simulink model "model_for_figure (EEE-13255's conflicted copy 2017-08-23)"  (R2016b)
settings: Solver=VariableStepAuto  StartTime=0.0  StopTime=5000  RelTol=1e-3
undefined symbols (not defined in the file or in its folder): sigbuilder_block
settings Model: Creator=utomo  LastModifiedBy=utomo

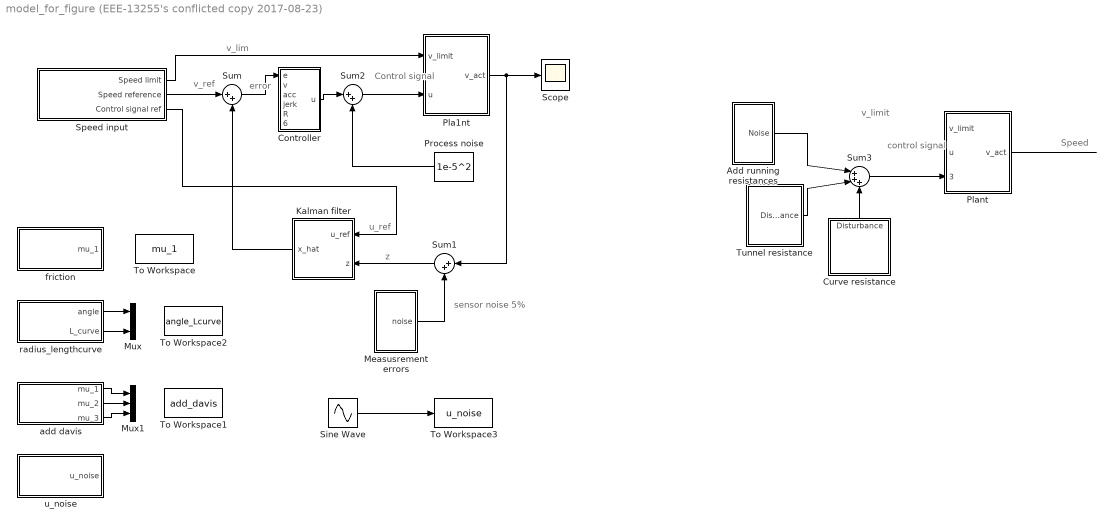
== system model_for_figure (EEE-13255's conflicted copy 2017-08-23) ==
  note: Speed
  note: control
      | signal
  note: v_limit
  note: sensor noise
      | 5%
  note: z
  note: error
  note: v_lim
  note: v_ref
  note: Control
      | signal
  note: u_ref
  Add running resistances : Subsystem
  Controller : Subsystem
  Curve resistance : Subsystem
  Kalman filter : Subsystem
  Measusrement errors : Subsystem
  Mux : Mux  Inputs=2
  Mux1 : Mux  Inputs=3
  Pla1nt : Subsystem
  Plant : Subsystem
  Process noise : Constant  Value=1e-5^2
  Scope : Scope
  Sine Wave : Sin  Amplitude=1e-5^2  Frequency=1/100  SampleTime=1
  Speed input : Subsystem  Tag=STV Subsys  LoadFcn=sigbuilder_block('load');  StartFcn=sigbuilder_block('start');  StopFcn=sigbuilder_block('stop');  ClipboardFcn=sigbuilder_block('clipboard');  mask(Sigbuilder block){tuvar=[0:10]}
      mask help: Simulink:masks:SigbuilderBlock_MD
      mask init:
      | if ~strcmp(get_param(bdroot(gcbh),'SimulationStatus'),'stopped') tuvar = sigbuilder_block('maskInit'); end
      settings: CopyFcn=sigbuilder_block('copy');  DeleteFcn=sigbuilder_block('delete');  ModelCloseFcn=sigbuilder_block('modelClose');  PreSaveFcn=sigbuilder_block('preSave');  PauseFcn=sigbuilder_block('pause');  ContinueFcn=sigbuilder_block('continue');  NameChangeFcn=sigbuilder_block('namechange');  OpenFcn=sigbuilder_block('open',[437.25 153 550.5 359.25 ]);  CloseFcn=sigbuilder_block('close');
      mask Display: plot(0, 0, 100, 100,[2, 2, 32, 32, 2], [68, 8, 8, 68, 68],[32, 2], [38, 38], [32, 19, 2],[53, 60, 44], [32, 17, 17, 2],[16, 16, 31, 31]);txt = getActiveGroup(gcbh);text(2, 100, txt,'verticalAlignment', 'top');
  Sum : Sum  Inputs=|++
  Sum1 : Sum  Inputs=|++
  Sum2 : Sum  Inputs=|++
  Sum3 : Sum  Inputs=|+++
  To Workspace : ToWorkspace  VariableName=mu_1  SampleTime=1
      settings: Save2DSignal=2-D array (concatenate along first dimension)
  To Workspace1 : ToWorkspace  VariableName=add_davis  SampleTime=1
      settings: Save2DSignal=2-D array (concatenate along first dimension)
  To Workspace2 : ToWorkspace  VariableName=angle_Lcurve  SampleTime=1
      settings: Save2DSignal=2-D array (concatenate along first dimension)
  To Workspace3 : ToWorkspace  VariableName=u_noise  SampleTime=1
      settings: Save2DSignal=2-D array (concatenate along first dimension)
  Tunnel resistance : Subsystem
  add davis : Subsystem  Tag=STV Subsys  LoadFcn=sigbuilder_block('load');  StartFcn=sigbuilder_block('start');  StopFcn=sigbuilder_block('stop');  ClipboardFcn=sigbuilder_block('clipboard');  mask(Sigbuilder block){tuvar=[0:10]}
      mask help: Simulink:masks:SigbuilderBlock_MD
      mask init:
      | if ~strcmp(get_param(bdroot(gcbh),'SimulationStatus'),'stopped') tuvar = sigbuilder_block('maskInit'); end
      settings: CopyFcn=sigbuilder_block('copy');  DeleteFcn=sigbuilder_block('delete');  ModelCloseFcn=sigbuilder_block('modelClose');  PreSaveFcn=sigbuilder_block('preSave');  PauseFcn=sigbuilder_block('pause');  ContinueFcn=sigbuilder_block('continue');  NameChangeFcn=sigbuilder_block('namechange');  OpenFcn=sigbuilder_block('open',[437.25 153 550.5 359.25 ]);  CloseFcn=sigbuilder_block('close');
      mask Display: plot(0, 0, 100, 100,[2, 2, 32, 32, 2], [68, 8, 8, 68, 68],[32, 2], [38, 38], [32, 19, 2],[53, 60, 44], [32, 17, 17, 2],[16, 16, 31, 31]);txt = getActiveGroup(gcbh);text(2, 100, txt,'verticalAlignment', 'top');
  "friction " : Subsystem  Tag=STV Subsys  LoadFcn=sigbuilder_block('load');  StartFcn=sigbuilder_block('start');  StopFcn=sigbuilder_block('stop');  ClipboardFcn=sigbuilder_block('clipboard');  mask(Sigbuilder block){tuvar=[0:10]}
      mask help: Simulink:masks:SigbuilderBlock_MD
      mask init:
      | if ~strcmp(get_param(bdroot(gcbh),'SimulationStatus'),'stopped') tuvar = sigbuilder_block('maskInit'); end
      settings: CopyFcn=sigbuilder_block('copy');  DeleteFcn=sigbuilder_block('delete');  ModelCloseFcn=sigbuilder_block('modelClose');  PreSaveFcn=sigbuilder_block('preSave');  PauseFcn=sigbuilder_block('pause');  ContinueFcn=sigbuilder_block('continue');  NameChangeFcn=sigbuilder_block('namechange');  OpenFcn=sigbuilder_block('open',[437.25 153 550.5 359.25 ]);  CloseFcn=sigbuilder_block('close');
      mask Display: plot(0, 0, 100, 100,[2, 2, 32, 32, 2], [68, 8, 8, 68, 68],[32, 2], [38, 38], [32, 19, 2],[53, 60, 44], [32, 17, 17, 2],[16, 16, 31, 31]);txt = getActiveGroup(gcbh);text(2, 100, txt,'verticalAlignment', 'top');
  radius_lengthcurve : Subsystem  Tag=STV Subsys  LoadFcn=sigbuilder_block('load');  StartFcn=sigbuilder_block('start');  StopFcn=sigbuilder_block('stop');  ClipboardFcn=sigbuilder_block('clipboard');  mask(Sigbuilder block){tuvar=[0:10]}
      mask help: Simulink:masks:SigbuilderBlock_MD
      mask init:
      | if ~strcmp(get_param(bdroot(gcbh),'SimulationStatus'),'stopped') tuvar = sigbuilder_block('maskInit'); end
      settings: CopyFcn=sigbuilder_block('copy');  DeleteFcn=sigbuilder_block('delete');  ModelCloseFcn=sigbuilder_block('modelClose');  PreSaveFcn=sigbuilder_block('preSave');  PauseFcn=sigbuilder_block('pause');  ContinueFcn=sigbuilder_block('continue');  NameChangeFcn=sigbuilder_block('namechange');  OpenFcn=sigbuilder_block('open',[416.25 111.75 550.5 359.25 ]);  CloseFcn=sigbuilder_block('close');
      mask Display: plot(0, 0, 100, 100,[2, 2, 32, 32, 2], [68, 8, 8, 68, 68],[32, 2], [38, 38], [32, 19, 2],[53, 60, 44], [32, 17, 17, 2],[16, 16, 31, 31]);txt = getActiveGroup(gcbh);text(2, 100, txt,'verticalAlignment', 'top');
  u_noise : Subsystem  Tag=STV Subsys  LoadFcn=sigbuilder_block('load');  StartFcn=sigbuilder_block('start');  StopFcn=sigbuilder_block('stop');  ClipboardFcn=sigbuilder_block('clipboard');  mask(Sigbuilder block){tuvar=[0:10]}
      mask help: Simulink:masks:SigbuilderBlock_MD
      mask init:
      | if ~strcmp(get_param(bdroot(gcbh),'SimulationStatus'),'stopped') tuvar = sigbuilder_block('maskInit'); end
      settings: CopyFcn=sigbuilder_block('copy');  DeleteFcn=sigbuilder_block('delete');  ModelCloseFcn=sigbuilder_block('modelClose');  PreSaveFcn=sigbuilder_block('preSave');  PauseFcn=sigbuilder_block('pause');  ContinueFcn=sigbuilder_block('continue');  NameChangeFcn=sigbuilder_block('namechange');  OpenFcn=sigbuilder_block('open',[437.25 153 550.5 359.25 ]);  CloseFcn=sigbuilder_block('close');
      mask Display: plot(0, 0, 100, 100,[2, 2, 32, 32, 2], [68, 8, 8, 68, 68],[32, 2], [38, 38], [32, 19, 2],[53, 60, 44], [32, 17, 17, 2],[16, 16, 31, 31]);txt = getActiveGroup(gcbh);text(2, 100, txt,'verticalAlignment', 'top');
  wires:
  Sum/1 -> Controller/1(e)
  Speed input/2(Speed reference) -> Sum/1
  Speed input/1(Speed limit) -> Pla1nt/1(v_limit)
  Pla1nt/1(v_act) -> Sum1/1, Scope/1
  Measusrement errors/1(noise) -> Sum1/2
  Sum1/1 -> Kalman filter/2(z)
  Kalman filter/1(x_hat) -> Sum/2
  Speed input/3(Control signal ref) -> Kalman filter/1(u_ref)
  Controller/1(u) -> Sum2/1
  Sum2/1 -> Pla1nt/2(u)
  Process noise/1 -> Sum2/2
  radius_lengthcurve/1(angle) -> Mux/1
  radius_lengthcurve/2(L_curve) -> Mux/2
  add davis/2(mu_2) -> Mux1/2
  add davis/3(mu_3) -> Mux1/3
  add davis/1(mu_1) -> Mux1/1
  Sine Wave/1 -> To Workspace3/1
  Sum3/1 -> Plant/3(disturbances)
  Add running resistances/1(Noise) -> Sum3/1
  Tunnel resistance/1(Disturbance) -> Sum3/2
  Curve resistance/1(Disturbance) -> Sum3/3
  ? -> Plant/1(v_limit)
  ? -> Plant/2(u)
  Plant/1(v_act) -> ?

== system model_for_figure (EEE-13255's conflicted copy 2017-08-23)/Add running resistances ==
  Gain : Gain
  Noise : Outport
  wires:
  ? -> Gain/1
  Gain/1 -> Noise/1

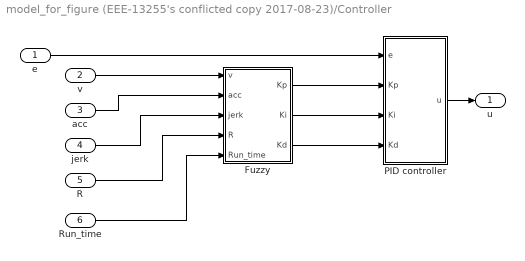
== system model_for_figure (EEE-13255's conflicted copy 2017-08-23)/Controller ==
  e : Inport
  v : Inport  Port=2
  acc : Inport  Port=3
  jerk : Inport  Port=4
  R : Inport  Port=5
  Run_time : Inport  Port=6
  Fuzzy : Subsystem
  PID controller : Subsystem
  u : Outport
  wires:
  e/1 -> PID controller/1(e)
  PID controller/1(u) -> u/1
  Fuzzy/1(Kp) -> PID controller/2(Kp)
  Fuzzy/2(Ki) -> PID controller/3(Ki)
  Fuzzy/3(Kd) -> PID controller/4(Kd)
  v/1 -> Fuzzy/1(v)
  acc/1 -> Fuzzy/2(acc)
  jerk/1 -> Fuzzy/3(jerk)
  R/1 -> Fuzzy/4(R)
  Run_time/1 -> Fuzzy/5(Run_time)

== system model_for_figure (EEE-13255's conflicted copy 2017-08-23)/Curve resistance ==
  Gain : Gain
  Disturbance : Outport
  wires:
  ? -> Gain/1
  Gain/1 -> Disturbance/1

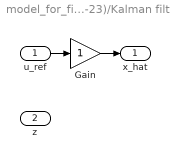
== system model_for_figure (EEE-13255's conflicted copy 2017-08-23)/Kalman filter ==
  u_ref : Inport
  z : Inport  Port=2
  Gain : Gain
  x_hat : Outport
  wires:
  u_ref/1 -> Gain/1
  Gain/1 -> x_hat/1

== system model_for_figure (EEE-13255's conflicted copy 2017-08-23)/Measusrement errors ==
  Gain : Gain
  noise : Outport
  wires:
  Gain/1 -> noise/1
  ? -> Gain/1

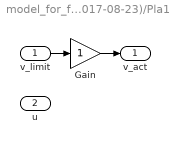
== system model_for_figure (EEE-13255's conflicted copy 2017-08-23)/Pla1nt ==
  v_limit : Inport
  u : Inport  Port=2
  Gain : Gain
  v_act : Outport
  wires:
  v_limit/1 -> Gain/1
  Gain/1 -> v_act/1

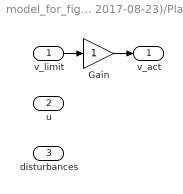
== system model_for_figure (EEE-13255's conflicted copy 2017-08-23)/Plant ==
  v_limit : Inport
  u : Inport  Port=2
  disturbances : Inport  Port=3
  Gain : Gain
  v_act : Outport
  wires:
  Gain/1 -> v_act/1
  v_limit/1 -> Gain/1

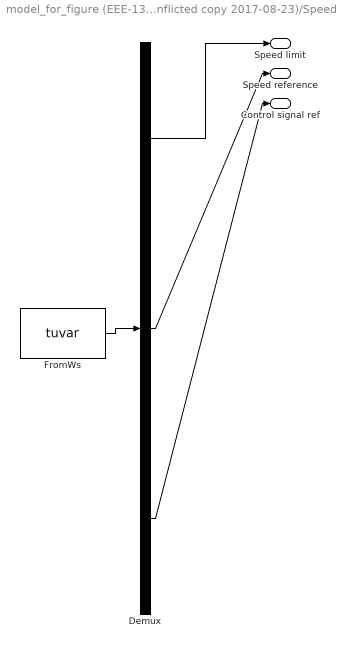
== system model_for_figure (EEE-13255's conflicted copy 2017-08-23)/Speed input ==
  Demux : Demux  Tag=STV Demux  Outputs=3
  FromWs : FromWorkspace  Tag=STV FromWs  VariableName=tuvar  SampleTime=0
      SigBuilderData=|
      | common.afterFinalStr = 'Extrapolate'
      | common.sampleTime = 0
      | dataSet.timeRange = [0 10]
      | dataSet.name = 'Group 1'
      | sbobj.Groups.Name = 'Group 1'
      | sbobj.Groups.Signals(1).Name = 'Speed limit'
      | sbobj.Groups.Signals(1).XData = [0 4 4 6 6 10]
      | sbobj.Groups.Signals(1).YData = [0 0 1 1 0 0]
      | sbobj.Groups.Signals(2).Name = 'Speed reference'
      | sbobj.Groups.Signals(2).XData = [0 10]
      | sbobj.Groups.Signals(2).YData = [0 0]
      | sbobj.Groups.Signals(3).Name = 'Control signal ref'
      | sbobj.Groups.Signals(3).XData = [0 10]
      | sbobj.Groups.Signals(3).YData = [0 0]
  Speed limit : Outport  Tag=STV Outport
  Speed reference : Outport  Tag=STV Outport  Port=2
  Control signal ref : Outport  Tag=STV Outport  Port=3
  wires:
  Demux/1 -> Speed limit/1
  FromWs/1 -> Demux/1
  Demux/2 -> Speed reference/1
  Demux/3 -> Control signal ref/1

== system model_for_figure (EEE-13255's conflicted copy 2017-08-23)/Tunnel resistance ==
  Gain : Gain
  Disturbance : Outport
  wires:
  Gain/1 -> Disturbance/1
  ? -> Gain/1

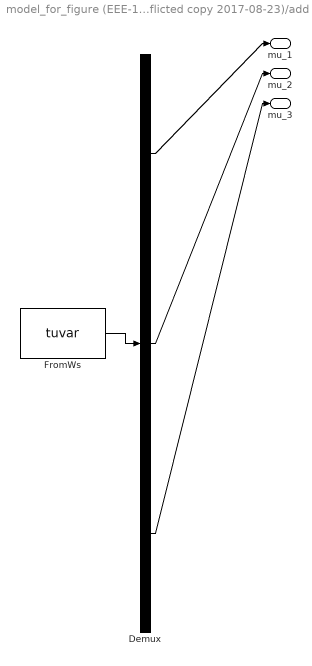
== system model_for_figure (EEE-13255's conflicted copy 2017-08-23)/add davis ==
  Demux : Demux  Tag=STV Demux  Outputs=3
  FromWs : FromWorkspace  Tag=STV FromWs  VariableName=tuvar
      SigBuilderData=|
      | common.afterFinalStr = 'Extrapolate'
      | common.sampleTime = '-1'
      | dataSet.timeRange = [0 5000]
      | dataSet.name = 'Group 1'
      | sbobj.Groups.Name = 'Group 1'
      | sbobj.Groups.Signals(1).Name = 'mu_1'
      | sbobj.Groups.Signals(1).XData = [0 500 500 1000 1500 2000 2000 2500 3000 3500 4000 4500 5000]
      | sbobj.Groups.Signals(1).YData = [1 0.7 0.9 1.1 1 1.2 0.8 0.9 0.9 1.1 1.05 0.9 1.1]
      | sbobj.Groups.Signals(2).Name = 'mu_2'
      | sbobj.Groups.Signals(2).XData = [0 500 500 1000 1500 2000 2000 2500 3000 3500 4000 4500 5000]
      | sbobj.Groups.Signals(2).YData = [0.9 1 0.9 1 0.8 1 1.1 0.7 1.2 0.9 1 1.1 0.9]
      | sbobj.Groups.Signals(3).Name = 'mu_3'
      | sbobj.Groups.Signals(3).XData = [0 500 500 1000 1500 2000 2000 2500 3000 3500 4000 4500 5000]
      | sbobj.Groups.Signals(3).YData = [0.7 0.8 1 0.8 1.1 0.8 1 1.05 1.1 1.2 0.8 0.9 0.99]
      | sbobj.Groups.TimeRange = [0 5000]
  mu_1 : Outport  Tag=STV Outport
  mu_2 : Outport  Tag=STV Outport  Port=2
  mu_3 : Outport  Tag=STV Outport  Port=3
  wires:
  Demux/1 -> mu_1/1
  FromWs/1 -> Demux/1
  Demux/2 -> mu_2/1
  Demux/3 -> mu_3/1

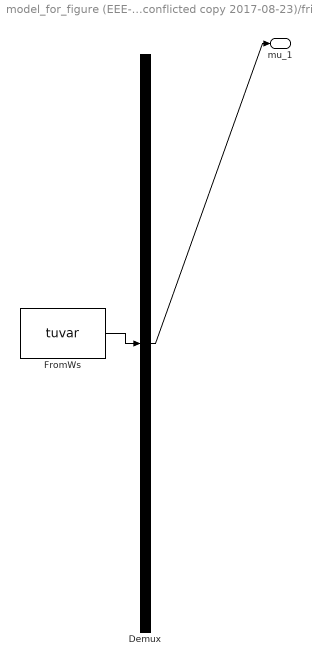
== system model_for_figure (EEE-13255's conflicted copy 2017-08-23)/friction  ==
  Demux : Demux  Tag=STV Demux  Outputs=1
  FromWs : FromWorkspace  Tag=STV FromWs  VariableName=tuvar
      SigBuilderData=|
      | common.afterFinalStr = 'Extrapolate'
      | common.sampleTime = '-1'
      | dataSet.timeRange = [0 5000]
      | dataSet.name = 'Group 1'
      | sbobj.Groups.Name = 'Group 1'
      | sbobj.Groups.Signals.Name = 'mu_1'
      | sbobj.Groups.Signals.XData = [0 3.24 500 1000 1500 2000 2000 2500 3000 3500 4000 4500 5000]
      | sbobj.Groups.Signals.YData = [0 0 0.1 0.385 0.6 0.25 0.05 0.305 0.9 0.8 0.7 0.2 0.499401197605]
      | sbobj.Groups.TimeRange = [0 5000]
  mu_1 : Outport  Tag=STV Outport
  wires:
  FromWs/1 -> Demux/1
  Demux/1 -> mu_1/1

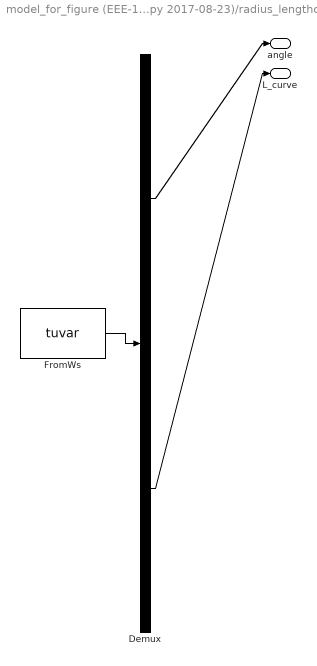
== system model_for_figure (EEE-13255's conflicted copy 2017-08-23)/radius_lengthcurve ==
  Demux : Demux  Tag=STV Demux  Outputs=2
  FromWs : FromWorkspace  Tag=STV FromWs  VariableName=tuvar
      SigBuilderData=|
      | common.afterFinalStr = 'Extrapolate'
      | common.sampleTime = '-1'
      | dataSet.timeRange = [0 5000]
      | dataSet.name = 'Group 1'
      | sbobj.Groups.Name = 'Group 1'
      | sbobj.Groups.Signals(1).Name = 'angle'
      | sbobj.Groups.Signals(1).XData = [0 3.24 101 101 300 300 3001 3001 4000 4000 4401 4401 4900 4900 5000]
      | sbobj.Groups.Signals(1).YData = [0 0 0 90 90 0 0 190 190 0 0 75 75 0 0]
      | sbobj.Groups.Signals(2).Name = 'L_curve'
      | sbobj.Groups.Signals(2).XData = [0 3.24 101 101 300 300 3001 3001 4000 4000 4401 4401 4900 4900 5000]
      | sbobj.Groups.Signals(2).YData = [0 0 0 200 200 0 0 1000 1000 0 0 500 500 0 0]
      | sbobj.Groups.TimeRange = [0 5000]
  angle : Outport  Tag=STV Outport
  L_curve : Outport  Tag=STV Outport  Port=2
  wires:
  Demux/1 -> angle/1
  FromWs/1 -> Demux/1
  Demux/2 -> L_curve/1

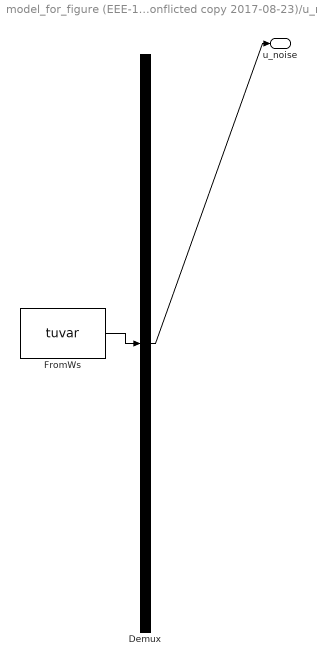
== system model_for_figure (EEE-13255's conflicted copy 2017-08-23)/u_noise ==
  Demux : Demux  Tag=STV Demux  Outputs=1
  FromWs : FromWorkspace  Tag=STV FromWs  VariableName=tuvar
      SigBuilderData=|
      | common.afterFinalStr = 'Extrapolate'
      | common.sampleTime = '-1'
      | dataSet.timeRange = [0 5000]
      | dataSet.name = 'Group 1'
      | sbobj.Groups.Name = 'Group 1'
      | sbobj.Groups.Signals.Name = 'u_noise'
      | sbobj.Groups.Signals.XData = [0 500 500 1000 1000 1500 1500 2000 2000 2500 2500 3000 3000 3500 3500 4000 4000 4500 4500 5000]
      | sbobj.Groups.Signals.YData = [0 1e-10 0 -1e-10 0 1e-10 0 -1e-10 0 1e-10 0 -1e-10 0 1e-10 0 -1e-10 0 1e-10 0 -1e-10]
      | sbobj.Groups.TimeRange = [0 5000]
  u_noise : Outport  Tag=STV Outport
  wires:
  Demux/1 -> u_noise/1
  FromWs/1 -> Demux/1

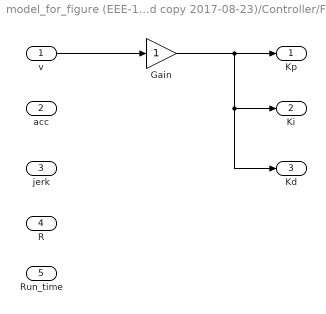
== system model_for_figure (EEE-13255's conflicted copy 2017-08-23)/Controller/Fuzzy ==
  v : Inport
  acc : Inport  Port=2
  jerk : Inport  Port=3
  R : Inport  Port=4
  Run_time : Inport  Port=5
  Gain : Gain
  Kp : Outport
  Ki : Outport  Port=2
  Kd : Outport  Port=3
  wires:
  v/1 -> Gain/1
  Gain/1 -> Kd/1, Ki/1, Kp/1

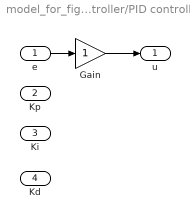
== system model_for_figure (EEE-13255's conflicted copy 2017-08-23)/Controller/PID controller ==
  e : Inport
  Kp : Inport  Port=2
  Ki : Inport  Port=3
  Kd : Inport  Port=4
  Gain : Gain
  u : Outport
  wires:
  Gain/1 -> u/1
  e/1 -> Gain/1
